simulink model "simulink_to_apollo"  (R2018b)
settings: Solver=VariableStepAuto  StartTime=0.0  StopTime=inf  RelTol=1e-3
model workspace (MAT data in the model file):
  SL_ROS_VariableLengthArrays_MaxSizes.CommonInfo.ArrayTruncateAction = 'EmitWarning'
  SL_ROS_VariableLengthArrays_MaxSizes.MsgTypeMap = containers.Map
  SL_ROS_VariableLengthArrays_MaxSizes.MsgTypeMap.serialization.keys = {'my_msgs/Header', 'sensor_msgs/PointCloud2', 'sensor_msgs/PointField'}
  SL_ROS_VariableLengthArrays_MaxSizes.MsgTypeMap.serialization.values{1}.PropertyName = 'ModuleName'
  SL_ROS_VariableLengthArrays_MaxSizes.MsgTypeMap.serialization.values{1}.DataType = 'uint8'
  SL_ROS_VariableLengthArrays_MaxSizes.MsgTypeMap.serialization.values{1}.MaxLength = 1
  SL_ROS_VariableLengthArrays_MaxSizes.MsgTypeMap.serialization.values{2}(1).PropertyName = 'Data'
  SL_ROS_VariableLengthArrays_MaxSizes.MsgTypeMap.serialization.values{2}(1).DataType = 'uint8'
  SL_ROS_VariableLengthArrays_MaxSizes.MsgTypeMap.serialization.values{2}(1).MaxLength = 128
  SL_ROS_VariableLengthArrays_MaxSizes.MsgTypeMap.serialization.values{2}(2).PropertyName = 'Fields'
  SL_ROS_VariableLengthArrays_MaxSizes.MsgTypeMap.serialization.values{2}(2).DataType = 'sensor_msgs/PointField'
  SL_ROS_VariableLengthArrays_MaxSizes.MsgTypeMap.serialization.values{2}(2).MaxLength = 4
  SL_ROS_VariableLengthArrays_MaxSizes.MsgTypeMap.serialization.values{3}.PropertyName = 'Name'
  SL_ROS_VariableLengthArrays_MaxSizes.MsgTypeMap.serialization.values{3}.DataType = 'uint8'
  SL_ROS_VariableLengthArrays_MaxSizes.MsgTypeMap.serialization.values{3}.MaxLength = 1
  SL_ROS_VariableLengthArrays_MaxSizes.MsgTypeMap.serialization.uniformity = 0
  SL_ROS_VariableLengthArrays_MaxSizes.MsgTypeMap.serialization.keyType = 'char'
  SL_ROS_VariableLengthArrays_MaxSizes.MsgTypeMap.serialization.valueType = 'any'
undefined symbols (not defined in the file): Brake, Count, Datatype, Fields, Fields_SL_Info, GearLocation, Header, Height, Name, Name_SL_Info, Offset, PointStep, RowStep, SteeringRate, SteeringTarget, Throttle, Width
libraries: robotlib x12
settings Model: Creator=mskim  LastModifiedBy=mskim

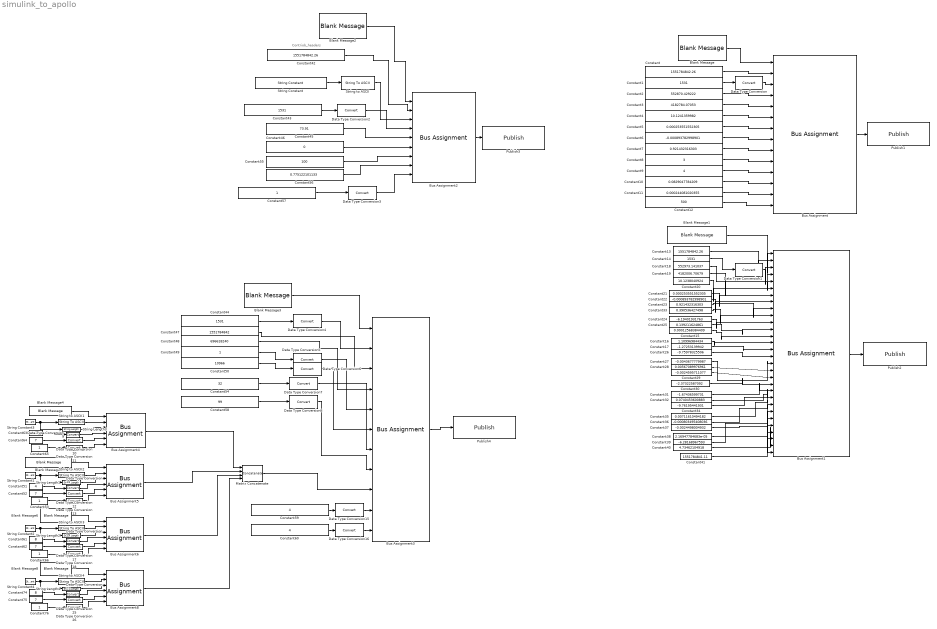
== system simulink_to_apollo ==
  note: Contriob_headers
  Blank Message : robotlib/Blank Message  messageClass=Message  entityType=my_msgs/Gps  messageType=my_msgs/Gps  SampleTime=inf
      settings: SourceProductBaseCode=RO
  Blank Message1 : robotlib/Blank Message  messageClass=Message  entityType=my_msgs/LocalizationEstimate  messageType=my_msgs/LocalizationEstimate  SampleTime=inf
      settings: SourceProductBaseCode=RO
  Blank Message2 : robotlib/Blank Message  messageClass=Message  entityType=my_msgs/ControlCommand  messageType=my_msgs/ControlCommand  SampleTime=inf
      settings: SourceProductBaseCode=RO
  Blank Message3 : robotlib/Blank Message  messageClass=Message  entityType=sensor_msgs/PointCloud2  messageType=sensor_msgs/PointCloud2  SampleTime=inf
      settings: SourceProductBaseCode=RO
  Blank Message{4..6,8} (4 alike) : robotlib/Blank Message  messageClass=Message  entityType=sensor_msgs/PointField  messageType=sensor_msgs/PointField  SampleTime=inf
      settings: SourceProductBaseCode=RO
  Bus Assignment : BusAssignment  AssignedSignals=Header.TimestampSec,Header.SequenceNum,Localization.Heading,Localization.Position.X,Localization.Position.Y,Localization.Position.Z,Localization.Orientation.Qx,Localization.Orientation.Qy,Localization.Orientation.Qz,Localization.Orientation.Qw,Localization.LinearVelocity.X,Localization.LinearVelocity.Y,Localization.LinearVelocity.Z
  Bus Assignment1 : BusAssignment  AssignedSignals=Header.TimestampSec,Header.SequenceNum,Pose.Position.X,Pose.Position.Y,Pose.Position.Z,Pose.Orientation.Qx,Pose.Orientation.Qy,Pose.Orientation.Qz,Pose.Orientation.Qw,Pose.LinearVelocity.X,Pose.LinearVelocity.Y,Pose.LinearVelocity.Z,Pose.LinearAccelration.X,Pose.LinearAccelration.Y,Pose.LinearAccelration.Z,Pose.AngularVelocity.X,Pose.AngularVelocity.Y,Pose.AngularVelocity.Z,Pose.Heading,Pose.LinearAccelerationVrf.X,Pose.LinearAccelerationVrf.Y,Pose.LinearAccelerationVrf.Z,Pose.AngularAccelerationVrf.X,Pose.AngularAccelerationVrf.Y,Pose.AngularAccelerationVrf.Z,Pose.EulerAngles.X,Pose.EulerAngles.Y,Pose.EulerAngles.Z,MeasurementTime
  Bus Assignment2 : BusAssignment  AssignedSignals=Header.TimestampSec,Header.ModuleName,Header.SequenceNum,Throttle,Brake,SteeringRate,SteeringTarget,GearLocation
  Bus Assignment3 : BusAssignment  AssignedSignals=Header.Seq,Header.Stamp.Sec,Header.Stamp.Nsec,Height,Width,PointStep,RowStep,Fields,Fields_SL_Info.CurrentLength,Fields_SL_Info.ReceivedLength
  Bus Assignment{4..6,8} (4 alike) : BusAssignment  AssignedSignals=Name,Name_SL_Info.CurrentLength,Offset,Datatype,Count
  Constant : Constant  Value=1551784842.26
  Constant{1,14,43..44} (4 alike) : Constant  Value=1531
  Constant10 : Constant  Value=0.0829047784209
  Constant11 : Constant  Value=0.000244081020355
  Constant12 : Constant  Value=500
  Constant13 : Constant  Value=1551784842.26
  Constant15 : Constant  Value=0.00012568384409
  Constant16 : Constant  Value=1.10996984434
  Constant17 : Constant  Value=-1.27253139942
  Constant18 : Constant  Value=552973.141037
  Constant19 : Constant  Value=4182006.70679
  Constant2 : Constant  Value=552870.429222
  Constant20 : Constant  Value=10.1238040924
  Constant21 : Constant  Value=0.000253551552305
  Constant22 : Constant  Value=-0.000893782998901
  Constant23 : Constant  Value=0.921432316303
  Constant24 : Constant  Value=-6.19401931763
  Constant25 : Constant  Value=0.139211624861
  Constant26 : Constant  Value=-9.75978325506
  Constant27 : Constant  Value=-0.0043677779987
  Constant28 : Constant  Value=0.00567089976961
  Constant29 : Constant  Value=-0.0024595711077
  Constant3 : Constant  Value=4182784.07053
  Constant30 : Constant  Value=-2.37322587092
  Constant31 : Constant  Value=-1.67436599731
  Constant32 : Constant  Value=0.0740453600883
  Constant33 : Constant  Value=0.390536427498
  Constant34 : Constant  Value=-9.76195441931
  Constant35 : Constant  Value=0.00711610494182
  Constant36 : Constant  Value=-0.000803495408036
  Constant37 : Constant  Value=-0.0024498004932
  Constant38 : Constant  Value=2.16947784683e-05
  Constant39 : Constant  Value=-6.28168967593
  Constant4 : Constant  Value=10.1241359982
  Constant40 : Constant  Value=4.73462104918
  Constant41 : Constant  Value=1551784841.11
  Constant42 : Constant  Value=1551784842.26
  Constant45 : Constant  Value=73.91
  Constant46 : Constant  Value=0
  Constant47 : Constant  Value=1551784842
  Constant48 : Constant  Value=696618240
  Constant{49,53,57,65..66,76} (6 alike) : Constant
  Constant5 : Constant  Value=0.000253551552305
  Constant50 : Constant  Value=10966
  Constant{9,51,59..60} (4 alike) : Constant  Value=4
  Constant{52,62,64,75} (4 alike) : Constant  Value=7
  Constant54 : Constant  Value=32
  Constant55 : Constant  Value=100
  Constant56 : Constant  Value=0.775122101133
  Constant58 : Constant  Value=99
  Constant6 : Constant  Value=-0.000893782998901
  Constant61 : Constant  Value=8
  Constant63 : Constant  Value=0
  Constant7 : Constant  Value=0.921432316303
  Constant74 : Constant  Value=8
  Constant8 : Constant  Value=3
  Data Type Conversion{,1..19,25..27} (23 alike) : DataTypeConversion
  Matrix Concatenate : Concatenate  NumInputs=4  Mode=Multidimensional array  ConcatenateDimension=2
  Publish1 : robotlib/Publish  topicSource=Specify your own  topic=/my_msgs/Gps  messageType=my_msgs/Gps  messageQueueLength=1
      settings: SourceProductBaseCode=RO
  Publish2 : robotlib/Publish  topicSource=Specify your own  topic=/my_msgs/LocalizationEstimate  messageType=my_msgs/LocalizationEstimate  messageQueueLength=1
      settings: SourceProductBaseCode=RO
  Publish3 : robotlib/Publish  topicSource=Specify your own  topic=/my_msgs/ControlCommand  messageType=my_msgs/ControlCommand  messageQueueLength=1
      settings: SourceProductBaseCode=RO
  Publish4 : robotlib/Publish  topicSource=Specify your own  topic=/sensor_msgs/PointCloud2  messageType=sensor_msgs/PointCloud2  messageQueueLength=1
      settings: SourceProductBaseCode=RO
  String Constant : StringConstant  String="\"control\""
  String Constant1 : StringConstant  String="\"y\""
  String Constant2 : StringConstant  String="\"z\""
  String Constant3 : StringConstant  String="\"x\""
  String Constant4 : StringConstant  String="\"intensity\""
  String Length{1..4} (4 alike) : StringLength
  String to ASCII{,1..4} (5 alike) : StringToASCII  MaximumLength=1
  wires:
  Constant4/1 -> Bus Assignment/6
  Data Type Conversion/1 -> Bus Assignment/3
  Constant6/1 -> Bus Assignment/8
  Constant12/1 -> Bus Assignment/14
  Constant9/1 -> Bus Assignment/11
  Constant5/1 -> Bus Assignment/7
  Constant7/1 -> Bus Assignment/9
  Constant1/1 -> Data Type Conversion/1
  Constant2/1 -> Bus Assignment/4
  Constant3/1 -> Bus Assignment/5
  Blank Message/1 -> Bus Assignment/1
  Bus Assignment/1 -> Publish1/1
  Constant8/1 -> Bus Assignment/10
  Constant11/1 -> Bus Assignment/13
  Constant10/1 -> Bus Assignment/12
  Constant/1 -> Bus Assignment/2
  Constant13/1 -> Bus Assignment1/2
  Constant18/1 -> Bus Assignment1/4
  Constant19/1 -> Bus Assignment1/5
  Constant21/1 -> Bus Assignment1/7
  Bus Assignment1/1 -> Publish2/1
  Blank Message1/1 -> Bus Assignment1/1
  Constant14/1 -> Data Type Conversion1/1
  Data Type Conversion1/1 -> Bus Assignment1/3
  Constant20/1 -> Bus Assignment1/6
  Constant22/1 -> Bus Assignment1/8
  Constant23/1 -> Bus Assignment1/9
  Constant33/1 -> Bus Assignment1/10
  Constant24/1 -> Bus Assignment1/11
  Constant25/1 -> Bus Assignment1/12
  Constant15/1 -> Bus Assignment1/13
  Constant16/1 -> Bus Assignment1/14
  Constant17/1 -> Bus Assignment1/15
  Constant26/1 -> Bus Assignment1/16
  Constant27/1 -> Bus Assignment1/17
  Constant28/1 -> Bus Assignment1/18
  Constant29/1 -> Bus Assignment1/19
  Constant30/1 -> Bus Assignment1/20
  Constant31/1 -> Bus Assignment1/21
  Constant32/1 -> Bus Assignment1/22
  Constant34/1 -> Bus Assignment1/23
  Constant35/1 -> Bus Assignment1/24
  Constant36/1 -> Bus Assignment1/25
  Constant37/1 -> Bus Assignment1/26
  Constant38/1 -> Bus Assignment1/27
  Constant39/1 -> Bus Assignment1/28
  Constant40/1 -> Bus Assignment1/29
  Constant41/1 -> Bus Assignment1/30
  Bus Assignment2/1 -> Publish3/1
  Blank Message2/1 -> Bus Assignment2/1
  Constant42/1 -> Bus Assignment2/2
  Constant43/1 -> Data Type Conversion2/1
  Constant45/1 -> Bus Assignment2/5
  Constant46/1 -> Bus Assignment2/6
  Constant55/1 -> Bus Assignment2/7
  Constant56/1 -> Bus Assignment2/8
  String to ASCII/1 -> Bus Assignment2/3
  String Constant/1 -> String to ASCII/1
  Data Type Conversion2/1 -> Bus Assignment2/4
  Constant57/1 -> Data Type Conversion3/1
  Data Type Conversion3/1 -> Bus Assignment2/9
  Blank Message3/1 -> Bus Assignment3/1
  Constant50/1 -> Data Type Conversion6/1
  Bus Assignment3/1 -> Publish4/1
  String Length3/1 -> Bus Assignment4/3
  Data Type Conversion8/1 -> Bus Assignment3/8
  Data Type Conversion7/1 -> Bus Assignment3/7
  Constant54/1 -> Data Type Conversion7/1
  Data Type Conversion6/1 -> Bus Assignment3/6
  Constant64/1 -> Data Type Conversion10/1
  Data Type Conversion5/1 -> Bus Assignment3/5
  Constant47/1 -> Bus Assignment3/3
  Data Type Conversion11/1 -> Bus Assignment4/6
  Data Type Conversion9/1 -> Bus Assignment4/4
  Constant63/1 -> Data Type Conversion9/1
  Blank Message4/1 -> Bus Assignment4/1
  Data Type Conversion10/1 -> Bus Assignment4/5
  String Constant3/1 -> String Length3/1, String to ASCII1/1
  String to ASCII1/1 -> Bus Assignment4/2
  Constant58/1 -> Data Type Conversion8/1
  Constant44/1 -> Data Type Conversion4/1
  Constant48/1 -> Bus Assignment3/4
  Constant49/1 -> Data Type Conversion5/1
  Data Type Conversion4/1 -> Bus Assignment3/2
  Constant65/1 -> Data Type Conversion11/1
  Bus Assignment4/1 -> Matrix Concatenate/1
  Constant59/1 -> Data Type Conversion15/1
  Constant60/1 -> Data Type Conversion16/1
  Constant53/1 -> Data Type Conversion13/1
  String Constant1/1 -> String Length1/1, String to ASCII2/1
  Data Type Conversion14/1 -> Bus Assignment5/4
  Constant52/1 -> Data Type Conversion12/1
  Data Type Conversion13/1 -> Bus Assignment5/6
  String Length1/1 -> Bus Assignment5/3
  String to ASCII2/1 -> Bus Assignment5/2
  Blank Message5/1 -> Bus Assignment5/1
  Constant51/1 -> Data Type Conversion14/1
  Data Type Conversion12/1 -> Bus Assignment5/5
  Constant66/1 -> Data Type Conversion18/1
  String Constant2/1 -> String Length2/1, String to ASCII3/1
  Data Type Conversion19/1 -> Bus Assignment6/4
  Constant62/1 -> Data Type Conversion17/1
  Data Type Conversion18/1 -> Bus Assignment6/6
  String Length2/1 -> Bus Assignment6/3
  String to ASCII3/1 -> Bus Assignment6/2
  Blank Message6/1 -> Bus Assignment6/1
  Constant61/1 -> Data Type Conversion19/1
  Data Type Conversion17/1 -> Bus Assignment6/5
  Matrix Concatenate/1 -> Bus Assignment3/9
  Data Type Conversion15/1 -> Bus Assignment3/10
  Data Type Conversion16/1 -> Bus Assignment3/11
  Bus Assignment5/1 -> Matrix Concatenate/2
  Bus Assignment6/1 -> Matrix Concatenate/3
  Constant76/1 -> Data Type Conversion26/1
  Data Type Conversion27/1 -> Bus Assignment8/4
  Bus Assignment8/1 -> Matrix Concatenate/4
  String to ASCII4/1 -> Bus Assignment8/2
  Data Type Conversion25/1 -> Bus Assignment8/5
  Constant74/1 -> Data Type Conversion27/1
  String Constant4/1 -> String Length4/1, String to ASCII4/1
  Blank Message8/1 -> Bus Assignment8/1
  String Length4/1 -> Bus Assignment8/3
  Data Type Conversion26/1 -> Bus Assignment8/6
  Constant75/1 -> Data Type Conversion25/1
